simulink model "ABS_FUZZYPID_Controller"  (R2014a)
settings: Solver=ode45  SolverMode=SingleTasking  StartTime=0  StopTime=10  FixedStep=0.001  RelTol=1e-3  AbsTol=1e-6
libraries: fuzblock x8, Solver_SF x1
settings Model: ExtModeTrigMode=oneshot  ExtModeArmWhenConnect=off  Creator=jhu  LastModifiedBy=AUS
settings DataIOCC: LimitDataPoints=off  SignalLoggingSaveFormat=ModelDataLogs  SignalLoggingName=sigsOut
settings OptimizationCC: BlockReduction=off  BooleanDataType=off
settings DebuggingCC: SaveWithParameterizedLinksMsg=none  UnderspecifiedInitializationDetection=Classic  SignalResolutionControl=TryResolveAllWithWarning  SolverPrmCheckMsg=none  MultiTaskDSMMsg=warning  MultiTaskCondExecSysMsg=none  FcnCallInpInsideContextMsg=EnableAllAsWarning  StateNameClashWarn=warning
settings HardwareCC: TargetUnknown=on
settings RTWCC: TemplateMakefile=grt_vc.tmf  IncludeERTFirstTime=on
settings GRTTargetCC: TargetFcnLib=ansi_tfl_tmw.mat  CombineOutputUpdateFcns=off  GRTInterface=on

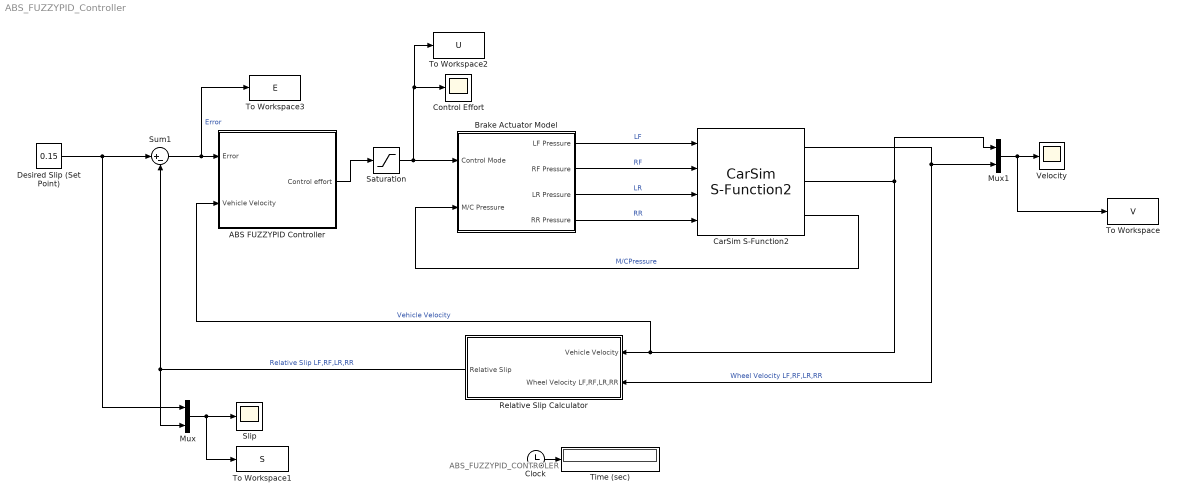
== system ABS_FUZZYPID_Controller ==
  note: ABS_FUZZYPID_CONTROLER
  ABS FUZZYPID Controller : Subsystem
  Brake Actuator Model : Subsystem
  CarSim S-Function2 : Solver_SF/CarSim S-Function2  Priority=1  VehicleCode=i_i  SIMFILE=simfile.sim
      settings: AttributesFormatString=Vehicle Code: %<VehicleCode>
  Clock : Clock
  Control Effort : Scope
      settings: ShowLegends=on  TimeRange=7  YMin=0  YMax=1  SaveName=ScopeData10  MaxDataPoints=50000
  "Desired Slip (Set Point) " : Constant  Value=0.15
  Mux : Mux  Inputs=2
  Mux1 : Mux  Inputs=2
  Relative Slip Calculator : Subsystem
  Saturation : Saturate  UpperLimit=1  LowerLimit=0
  Slip : Scope
      settings: TimeRange=6  YMin=0  YMax=1  MaxDataPoints=50000
  Sum1 : Sum  Inputs=|+-
  Time (sec) : Display
      settings: Format=bank  Decimation=100
  To Workspace : ToWorkspace  VariableName=V  SaveFormat=Timeseries  SampleTime=0.002
  To Workspace1 : ToWorkspace  VariableName=S  SaveFormat=Timeseries  SampleTime=0.002
  To Workspace2 : ToWorkspace  VariableName=U  SaveFormat=Timeseries  SampleTime=0.002
  To Workspace3 : ToWorkspace  VariableName=E  SaveFormat=Timeseries  SampleTime=0.002
  Velocity : Scope
      settings: ShowLegends=on  YMax=65  MaxDataPoints=50000
  wires:
  Clock/1 -> Time (sec)/1
  Brake Actuator Model/1(LF Pressure) -> CarSim S-Function2/1  "LF"
  Brake Actuator Model/2(RF Pressure) -> CarSim S-Function2/2  "RF"
  Brake Actuator Model/3(LR Pressure) -> CarSim S-Function2/3  "LR"
  Brake Actuator Model/4(RR Pressure) -> CarSim S-Function2/4  "RR"
  CarSim S-Function2/3 -> Brake Actuator Model/2(M/C Pressure)  "M/CPressure"
  "Desired Slip (Set Point) "/1 -> Sum1/1, Mux/1
  Mux/1 -> To Workspace1/1, Slip/1
  Relative Slip Calculator/1(Relative Slip) -> Sum1/2, Mux/2  "Relative Slip LF,RF,LR,RR"
  CarSim S-Function2/2 -> ABS FUZZYPID Controller/2(Vehicle Velocity), Relative Slip Calculator/1(Vehicle Velocity), Mux1/1  "Vehicle Velocity"
  CarSim S-Function2/1 -> Relative Slip Calculator/2(Wheel Velocity LF,RF,LR,RR), Mux1/2  "Wheel Velocity LF,RF,LR,RR"
  ABS FUZZYPID Controller/1(Control effort) -> Saturation/1
  Sum1/1 -> To Workspace3/1, ABS FUZZYPID Controller/1(Error)  "Error"
  Saturation/1 -> To Workspace2/1, Control Effort/1, Brake Actuator Model/1(Control Mode)
  Mux1/1 -> To Workspace/1, Velocity/1

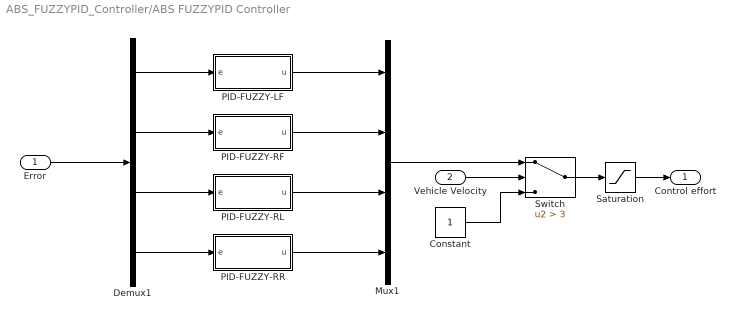
== system ABS_FUZZYPID_Controller/ABS FUZZYPID Controller ==
  Error : Inport
  Vehicle Velocity : Inport  Port=2
  Constant : Constant
  Demux1 : Demux
  Mux1 : Mux
  PID-FUZZY-LF : Subsystem
  PID-FUZZY-RF : Subsystem
  PID-FUZZY-RL : Subsystem
  PID-FUZZY-RR : Subsystem
  Saturation : Saturate  UpperLimit=1  LowerLimit=0
  Switch : Switch  Criteria=u2 > Threshold  Threshold=3
  Control effort : Outport
  wires:
  Error/1 -> Demux1/1
  Demux1/1 -> PID-FUZZY-LF/1(e)
  PID-FUZZY-LF/1(u) -> Mux1/1
  Demux1/2 -> PID-FUZZY-RF/1(e)
  PID-FUZZY-RF/1(u) -> Mux1/2
  Demux1/3 -> PID-FUZZY-RL/1(e)
  PID-FUZZY-RL/1(u) -> Mux1/3
  Demux1/4 -> PID-FUZZY-RR/1(e)
  PID-FUZZY-RR/1(u) -> Mux1/4
  Vehicle Velocity/1 -> Switch/2
  Constant/1 -> Switch/3
  Mux1/1 -> Switch/1
  Switch/1 -> Saturation/1
  Saturation/1 -> Control effort/1

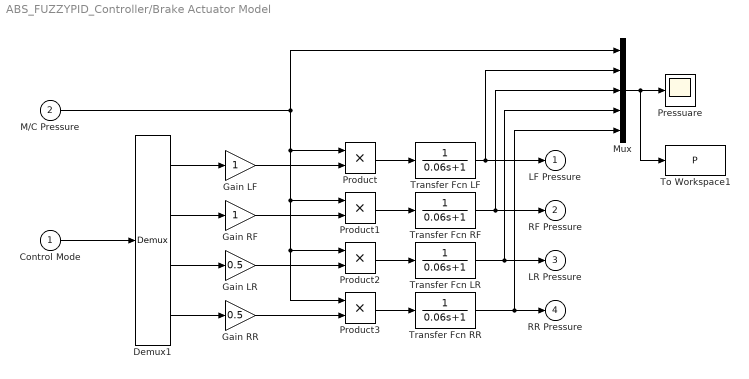
== system ABS_FUZZYPID_Controller/Brake Actuator Model ==
  Control Mode : Inport
  M/C Pressure : Inport  Port=2
  Demux1 : Demux
  Gain LF : Gain  SaturateOnIntegerOverflow=on  OutDataTypeStr=Inherit: Same as input  ParamDataTypeStr=Inherit: Same as input
  Gain LR : Gain  Gain=0.5  SaturateOnIntegerOverflow=on  OutDataTypeStr=Inherit: Same as input  ParamDataTypeStr=Inherit: Same as input
  Gain RF : Gain  SaturateOnIntegerOverflow=on  OutDataTypeStr=Inherit: Same as input  ParamDataTypeStr=Inherit: Same as input
  Gain RR : Gain  Gain=0.5  SaturateOnIntegerOverflow=on  OutDataTypeStr=Inherit: Same as input  ParamDataTypeStr=Inherit: Same as input
  Mux : Mux  Inputs=5
  Pressuare : Scope
      settings: ShowLegends=on  SaveName=ScopeData9
  Product{,1..3} (4 alike) : Product  SaturateOnIntegerOverflow=on  InputSameDT=on  OutDataTypeStr=Inherit: Same as first input
  To Workspace1 : ToWorkspace  VariableName=P  SaveFormat=Timeseries  SampleTime=0.002
  Transfer Fcn LF : TransferFcn  Denominator=[0.06 1]
  Transfer Fcn LR : TransferFcn  Denominator=[0.06 1]
  Transfer Fcn RF : TransferFcn  Denominator=[0.06 1]
  Transfer Fcn RR : TransferFcn  Denominator=[0.06 1]
  LF Pressure : Outport  InitialOutput=0
  RF Pressure : Outport  Port=2  InitialOutput=0
  LR Pressure : Outport  Port=3  InitialOutput=0
  RR Pressure : Outport  Port=4  InitialOutput=0
  wires:
  Control Mode/1 -> Demux1/1
  Gain LF/1 -> Product/2
  Gain RF/1 -> Product1/2
  Gain LR/1 -> Product2/2
  Gain RR/1 -> Product3/2
  M/C Pressure/1 -> Product/1, Product1/1, Product2/1, Product3/1, Mux/1
  Product/1 -> Transfer Fcn LF/1
  Product1/1 -> Transfer Fcn RF/1
  Product2/1 -> Transfer Fcn LR/1
  Product3/1 -> Transfer Fcn RR/1
  Demux1/1 -> Gain LF/1
  Demux1/2 -> Gain RF/1
  Demux1/3 -> Gain LR/1
  Demux1/4 -> Gain RR/1
  Transfer Fcn LF/1 -> Mux/2, LF Pressure/1
  Transfer Fcn RF/1 -> Mux/3, RF Pressure/1
  Transfer Fcn LR/1 -> Mux/4, LR Pressure/1
  Mux/1 -> To Workspace1/1, Pressuare/1
  Transfer Fcn RR/1 -> Mux/5, RR Pressure/1

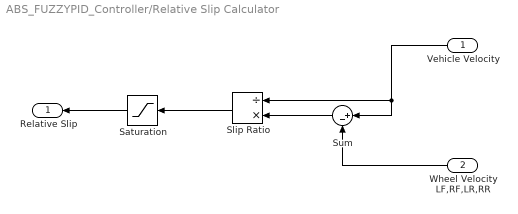
== system ABS_FUZZYPID_Controller/Relative Slip Calculator ==
  Vehicle Velocity : Inport
  Wheel Velocity LF,RF,LR,RR : Inport  Port=2
  Saturation : Saturate  UpperLimit=1  LowerLimit=0
  Slip Ratio : Product  Inputs=/*  SaturateOnIntegerOverflow=on  InputSameDT=on  OutDataTypeStr=Inherit: Same as first input
  Sum : Sum  Inputs=|+-
  Relative Slip : Outport
  wires:
  Vehicle Velocity/1 -> Slip Ratio/1, Sum/1
  Wheel Velocity LF,RF,LR,RR/1 -> Sum/2
  Sum/1 -> Slip Ratio/2
  Slip Ratio/1 -> Saturation/1
  Saturation/1 -> Relative Slip/1

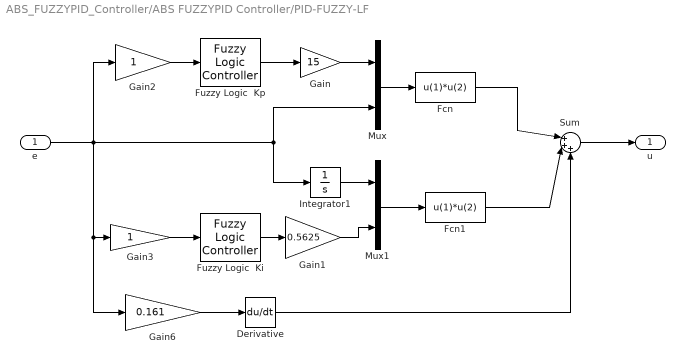
== system ABS_FUZZYPID_Controller/ABS FUZZYPID Controller/PID-FUZZY-LF ==
  e : Inport
  Derivative : Derivative
  Fcn : Fcn  Expr=u(1)*u(2)
  Fcn1 : Fcn  Expr=u(1)*u(2)
  Fuzzy Logic  Ki : fuzblock/Fuzzy Logic  Controller  fis='ABS_FUZZY-LOGIC-0.15.fis'
  Fuzzy Logic  Kp : fuzblock/Fuzzy Logic  Controller  fis='ABS_FUZZY-LOGIC-0.15.fis'
  Gain : Gain  Gain=15
  Gain1 : Gain  Gain=0.5625
  Gain2 : Gain
  Gain3 : Gain
  Gain6 : Gain  Gain=0.161
  Integrator1 : Integrator
  Mux : Mux  Inputs=2
  Mux1 : Mux  Inputs=2
  Sum : Sum  Inputs=|+++
  u : Outport
  wires:
  Fcn1/1 -> Sum/2
  Sum/1 -> u/1
  Fuzzy Logic  Kp/1 -> Gain/1
  Mux/1 -> Fcn/1
  Fcn/1 -> Sum/1
  Fuzzy Logic  Ki/1 -> Gain1/1
  Mux1/1 -> Fcn1/1
  Integrator1/1 -> Mux1/1
  Gain/1 -> Mux/1
  Gain1/1 -> Mux1/2
  e/1 -> Integrator1/1, Mux/2, Gain2/1, Gain6/1, Gain3/1
  Gain2/1 -> Fuzzy Logic  Kp/1
  Gain3/1 -> Fuzzy Logic  Ki/1
  Derivative/1 -> Sum/3
  Gain6/1 -> Derivative/1

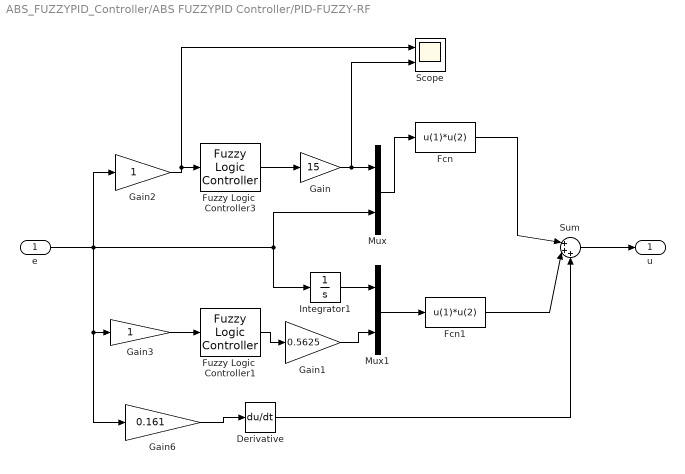
== system ABS_FUZZYPID_Controller/ABS FUZZYPID Controller/PID-FUZZY-RF ==
  e : Inport
  Derivative : Derivative
  Fcn : Fcn  Expr=u(1)*u(2)
  Fcn1 : Fcn  Expr=u(1)*u(2)
  Fuzzy Logic  Controller1 : fuzblock/Fuzzy Logic  Controller  fis='ABS_FUZZY-LOGIC-0.15.fis'
  Fuzzy Logic  Controller3 : fuzblock/Fuzzy Logic  Controller  fis='ABS_FUZZY-LOGIC-0.15.fis'
  Gain : Gain  Gain=15
  Gain1 : Gain  Gain=0.5625
  Gain2 : Gain
  Gain3 : Gain
  Gain6 : Gain  Gain=0.161
  Integrator1 : Integrator
  Mux : Mux  Inputs=2
  Mux1 : Mux  Inputs=2
  Scope : Scope  NumInputPorts=2
      settings: YMin=-5~-5  YMax=5~5  SaveName=ScopeData8
  Sum : Sum  Inputs=|+++
  u : Outport
  wires:
  Fcn1/1 -> Sum/2
  Sum/1 -> u/1
  Fuzzy Logic  Controller3/1 -> Gain/1
  Mux/1 -> Fcn/1
  Fcn/1 -> Sum/1
  Fuzzy Logic  Controller1/1 -> Gain1/1
  Mux1/1 -> Fcn1/1
  Integrator1/1 -> Mux1/1
  Gain/1 -> Scope/2, Mux/1
  Gain1/1 -> Mux1/2
  e/1 -> Integrator1/1, Mux/2, Gain2/1, Gain6/1, Gain3/1
  Gain2/1 -> Fuzzy Logic  Controller3/1, Scope/1
  Gain3/1 -> Fuzzy Logic  Controller1/1
  Derivative/1 -> Sum/3
  Gain6/1 -> Derivative/1

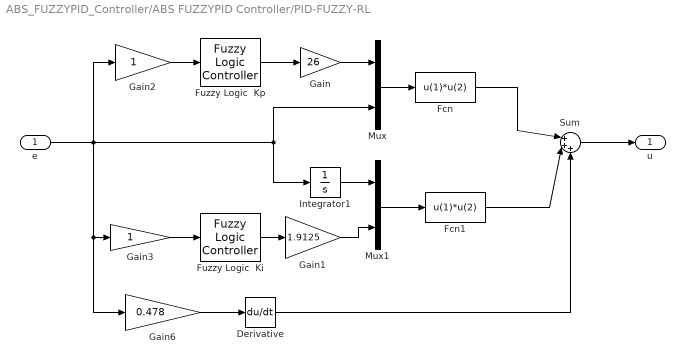
== system ABS_FUZZYPID_Controller/ABS FUZZYPID Controller/PID-FUZZY-RL ==
  e : Inport
  Derivative : Derivative
  Fcn : Fcn  Expr=u(1)*u(2)
  Fcn1 : Fcn  Expr=u(1)*u(2)
  Fuzzy Logic  Ki : fuzblock/Fuzzy Logic  Controller  fis='ABS_FUZZY-LOGIC-0.15.fis'
  Fuzzy Logic  Kp : fuzblock/Fuzzy Logic  Controller  fis='ABS_FUZZY-LOGIC-0.15.fis'
  Gain : Gain  Gain=26
  Gain1 : Gain  Gain=1.9125
  Gain2 : Gain
  Gain3 : Gain
  Gain6 : Gain  Gain=0.478
  Integrator1 : Integrator
  Mux : Mux  Inputs=2
  Mux1 : Mux  Inputs=2
  Sum : Sum  Inputs=|+++
  u : Outport
  wires:
  Fcn1/1 -> Sum/2
  Sum/1 -> u/1
  Fuzzy Logic  Kp/1 -> Gain/1
  Mux/1 -> Fcn/1
  Fcn/1 -> Sum/1
  Fuzzy Logic  Ki/1 -> Gain1/1
  Mux1/1 -> Fcn1/1
  Integrator1/1 -> Mux1/1
  Gain/1 -> Mux/1
  Gain1/1 -> Mux1/2
  e/1 -> Integrator1/1, Mux/2, Gain2/1, Gain6/1, Gain3/1
  Gain2/1 -> Fuzzy Logic  Kp/1
  Gain3/1 -> Fuzzy Logic  Ki/1
  Derivative/1 -> Sum/3
  Gain6/1 -> Derivative/1

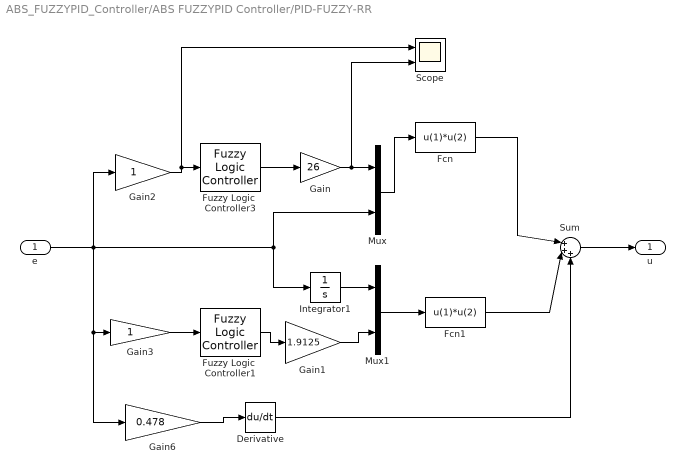
== system ABS_FUZZYPID_Controller/ABS FUZZYPID Controller/PID-FUZZY-RR ==
  e : Inport
  Derivative : Derivative
  Fcn : Fcn  Expr=u(1)*u(2)
  Fcn1 : Fcn  Expr=u(1)*u(2)
  Fuzzy Logic  Controller1 : fuzblock/Fuzzy Logic  Controller  fis='ABS_FUZZY-LOGIC-0.15.fis'
  Fuzzy Logic  Controller3 : fuzblock/Fuzzy Logic  Controller  fis='ABS_FUZZY-LOGIC-0.15.fis'
  Gain : Gain  Gain=26
  Gain1 : Gain  Gain=1.9125
  Gain2 : Gain
  Gain3 : Gain
  Gain6 : Gain  Gain=0.478
  Integrator1 : Integrator
  Mux : Mux  Inputs=2
  Mux1 : Mux  Inputs=2
  Scope : Scope  NumInputPorts=2
      settings: YMin=-5~-5  YMax=5~5  SaveName=ScopeData8
  Sum : Sum  Inputs=|+++
  u : Outport
  wires:
  Fcn1/1 -> Sum/2
  Sum/1 -> u/1
  Fuzzy Logic  Controller3/1 -> Gain/1
  Mux/1 -> Fcn/1
  Fcn/1 -> Sum/1
  Fuzzy Logic  Controller1/1 -> Gain1/1
  Mux1/1 -> Fcn1/1
  Integrator1/1 -> Mux1/1
  Gain/1 -> Scope/2, Mux/1
  Gain1/1 -> Mux1/2
  e/1 -> Integrator1/1, Mux/2, Gain2/1, Gain6/1, Gain3/1
  Gain2/1 -> Fuzzy Logic  Controller3/1, Scope/1
  Gain3/1 -> Fuzzy Logic  Controller1/1
  Derivative/1 -> Sum/3
  Gain6/1 -> Derivative/1
